simulink model "FinalCircuit"  (R2021b)
settings: Solver=ode4  StartTime=0.0  StopTime=2e-3  FixedStep=5e-10  RelTol=1e-3
values from neighbouring files (symbols this model uses):
  C = D/fs*(Vc-Vbat)/Rout/delVc    (= 1.03597563342e-05)    [Script.m]
  C2 = D2/fs*(Vc2-Vbat2)/Rout2/delVc2    (= 2.79316389763e-06)    [Script.m]
  fs = 250e3    (= 250000)    [Script.m]
  Gcinf = (abs(evalfr(Tuiind,1i*2*pi*fc)))/sqrt(1+(wLv/2/pi/fc)^2)/abs(evalfr(Gfilter,1i*2*pi*fc))    [Script.m]
  Gcinf2 = (abs(evalfr(Tuiind2,1i*2*pi*fc)))/sqrt(1+(wLv2/2/pi/fc)^2)/abs(evalfr(Gfilter,1i*2*pi*fc))    [Script.m]
  Lm = Vc*Dp/delIlm/fs    (= 0.000738946619669)    [Script.m]
  Lm2 = Vc2*Dp2/delIlm2/fs    (= 0.00253168682241)    [Script.m]
  Rin = 100e-3    (= 0.1)    [Script.m]
  Rout = Rin    (= 0.1)    [Script.m]
  Rsense = 5/0.2    (= 25)    [Script.m]
  Rsense2 = 5/0.1    (= 50)    [Script.m]
  Vbat = 3.7    [Script.m]
  Vin = 3.7    [Script.m]
  Vm = 5    [Script.m]
  wLv = 2*pi*fc*tan(75*pi/180)    [Script.m]
  wLv2 = 2*pi*fc*tan(60*pi/180)    [Script.m]
  wpfilter = 2*pi*30e3    (= 188495.559215)    [Script.m]
  wpfilter2 = 2*pi*10e3    (= 62831.8530718)    [Script.m]
libraries: spsCurrentMeasurementLib x25, spsVoltageMeasurementLib x18, spsSeriesRLCBranchLib x12, spsMosfetLib x9, spsLinearTransformerLib x4, simulink x4, spsDCVoltageSourceLib x4, spsDiodeLib x2, spspowerguiLib x2, spsControlledCurrentSourceLib x1
settings Model: SimulationMode=rapid-accelerator  Creator=ee3210698  LastModifiedBy=ee3210698

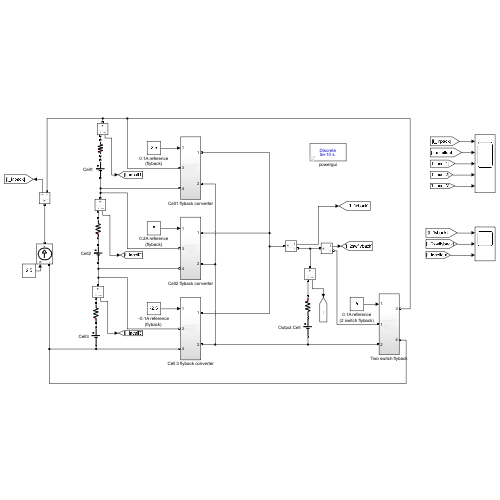
[thumbnail: Simulink's stored preview of the top-level diagram]
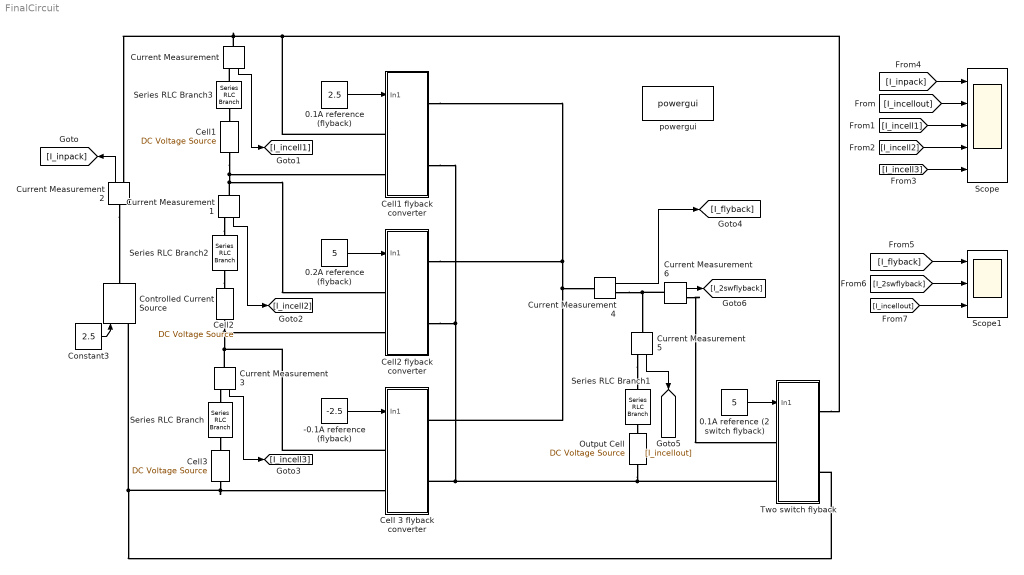
== system FinalCircuit ==
  "-0.1A reference (flyback) " : Constant  Value=-2.5
  0.1A reference (2 switch flyback) : Constant  Value=5
  0.1A reference (flyback) : Constant  Value=2.5
  0.2A reference (flyback) : Constant  Value=5
  Cell 3 flyback converter : Subsystem
  Cell1 : spsDCVoltageSourceLib/DC Voltage Source  Amplitude=Vin  Measurements=None
  Cell1 flyback converter : Subsystem
  Cell2 : spsDCVoltageSourceLib/DC Voltage Source  Amplitude=Vin  Measurements=None
  Cell2 flyback converter : Subsystem
  Cell3 : spsDCVoltageSourceLib/DC Voltage Source  Amplitude=Vin  Measurements=None
  Constant3 : Constant  Value=2.5
  Controlled Current Source : spsControlledCurrentSourceLib/Controlled Current Source  Initialize=on  Source_Type=DC  Amplitude=2.5  Phase=0  Frequency=0  Measurements=None
  Current Measurement{,1..6} (7 alike) : spsCurrentMeasurementLib/Current Measurement  PhasorSimulation=off  OutputType=Complex  PSBequivalent=0
  Output Cell : spsDCVoltageSourceLib/DC Voltage Source  Amplitude=Vbat  Measurements=None
  Scope : Scope  NumInputPorts=5
  Scope1 : Scope  NumInputPorts=3
  Series RLC Branch : spsSeriesRLCBranchLib/Series RLC Branch  LConnTagsString=__new0  RConnTagsString=__new0  BranchType=R  Resistance=Rin  Inductance=1e-3  SetiL0=off  InitialCurrent=0  Capacitance=1e-6  Setx0=off  InitialVoltage=0  Measurements=None
  Series RLC Branch1 : spsSeriesRLCBranchLib/Series RLC Branch  LConnTagsString=__new0  RConnTagsString=__new0  BranchType=R  Resistance=Rout  Inductance=1e-3  SetiL0=off  InitialCurrent=0  Capacitance=1e-6  Setx0=off  InitialVoltage=0  Measurements=None
  Series RLC Branch2 : spsSeriesRLCBranchLib/Series RLC Branch  LConnTagsString=__new0  RConnTagsString=__new0  BranchType=R  Resistance=Rin  Inductance=1e-3  SetiL0=off  InitialCurrent=0  Capacitance=1e-6  Setx0=off  InitialVoltage=0  Measurements=None
  Series RLC Branch3 : spsSeriesRLCBranchLib/Series RLC Branch  LConnTagsString=__new0  RConnTagsString=__new0  BranchType=R  Resistance=Rin  Inductance=1e-3  SetiL0=off  InitialCurrent=0  Capacitance=1e-6  Setx0=off  InitialVoltage=0  Measurements=None
  Two switch flyback : Subsystem
  powergui : spspowerguiLib/powergui  Priority=1  SimulationMode=Discrete  SampleTime=5e-10  frequency=60  Iterations=50  frequencyindice=0  Pbase=100e6  ErrMax=1e-4  UnitsV=kV  UnitsW=MW  buscounter=0  FunctionMessages=off  echomessages=off  EnableUseOfTLC=off  CurrentSourceSwitches=off  DisableSnubberDevices=off  DisableRonSwitches=off  DisableVfSwitches=off  DisplayEquations=off  AutomaticDiscreteSolvers=off  SolverType=Tustin/Backward Euler (TBE)  Interpol=off  ExternalGateDelay=off  methode=off  Ts=100  x0status=blocks  SPID=on  SwTol=0  HookPort=off  NonlinearTolerance=1e-4  nMaxIteration=100  ContinueOnMaxIteration=off  RestoreLinks=warning  ResistiveCurrentMeasurement=off  Frange=[0:2:500]  Ylog=off  Xlog=on  ShowGrid=off  save=off  variable=ZData  structure=0  ZoomFFT=off  StartTime=0.0  cycles=1  DisplayStyle=1  fundamental=60  FreqAxis=off  MaxFrequency=1000  frequencyindicesteady=1  RmsSteady=1  display=off
  wires:
  "-0.1A reference (flyback) "/1 -> Cell 3 flyback converter/1(In1)
  0.2A reference (flyback)/1 -> Cell2 flyback converter/1(In1)
  0.1A reference (flyback)/1 -> Cell1 flyback converter/1(In1)
  Current Measurement2/1 -> [I_inpack]
  Current Measurement1/1 -> [I_incell2]
  Current Measurement3/1 -> [I_incell3]
  Current Measurement4/1 -> [I_flyback]
  [I_incellout] -> Scope/2
  [I_incell1] -> Scope/3
  [I_incell2] -> Scope/4
  [I_incell3] -> Scope/5
  [I_inpack] -> Scope/1
  Constant3/1 -> Controlled Current Source/1
  Current Measurement/1 -> [I_incell1]
  0.1A reference (2 switch flyback)/1 -> Two switch flyback/1(In1)
  Current Measurement5/1 -> [I_incellout]
  [I_flyback] -> Scope1/1
  Current Measurement6/1 -> [I_2swflyback]
  [I_2swflyback] -> Scope1/2
  [I_incellout] -> Scope1/3
  connections:
  Cell3/LConn1 -- Cell 3 flyback converter/LConn2 -- Two switch flyback/RConn2 -- Controlled Current Source/LConn1
  Series RLC Branch/LConn1 -- Cell3/RConn1
  Series RLC Branch1/RConn1 -- Output Cell/RConn1
  Output Cell/LConn1 -- Cell1 flyback converter/RConn2 -- Cell2 flyback converter/RConn2 -- Cell 3 flyback converter/RConn2 -- Two switch flyback/LConn2
  Series RLC Branch2/LConn1 -- Cell2/RConn1
  Cell2/LConn1 -- Cell 3 flyback converter/LConn1 -- Current Measurement3/LConn1 -- Cell2 flyback converter/LConn2
  Cell1/LConn1 -- Cell2 flyback converter/LConn1 -- Current Measurement1/LConn1 -- Cell1 flyback converter/LConn2
  Series RLC Branch3/LConn1 -- Cell1/RConn1
  Cell1 flyback converter/LConn1 -- Current Measurement2/RConn1 -- Current Measurement/LConn1 -- Two switch flyback/RConn1
  Current Measurement2/LConn1 -- Controlled Current Source/RConn1
  Cell1 flyback converter/RConn1 -- Cell 3 flyback converter/RConn1 -- Current Measurement4/LConn1 -- Cell2 flyback converter/RConn1
  Current Measurement4/RConn1 -- Current Measurement6/LConn1 -- Current Measurement5/LConn1
  Series RLC Branch3/RConn1 -- Current Measurement/RConn1
  Current Measurement1/RConn1 -- Series RLC Branch2/RConn1
  Current Measurement3/RConn1 -- Series RLC Branch/RConn1
  Current Measurement5/RConn1 -- Series RLC Branch1/LConn1
  Current Measurement6/RConn1 -- Two switch flyback/LConn1

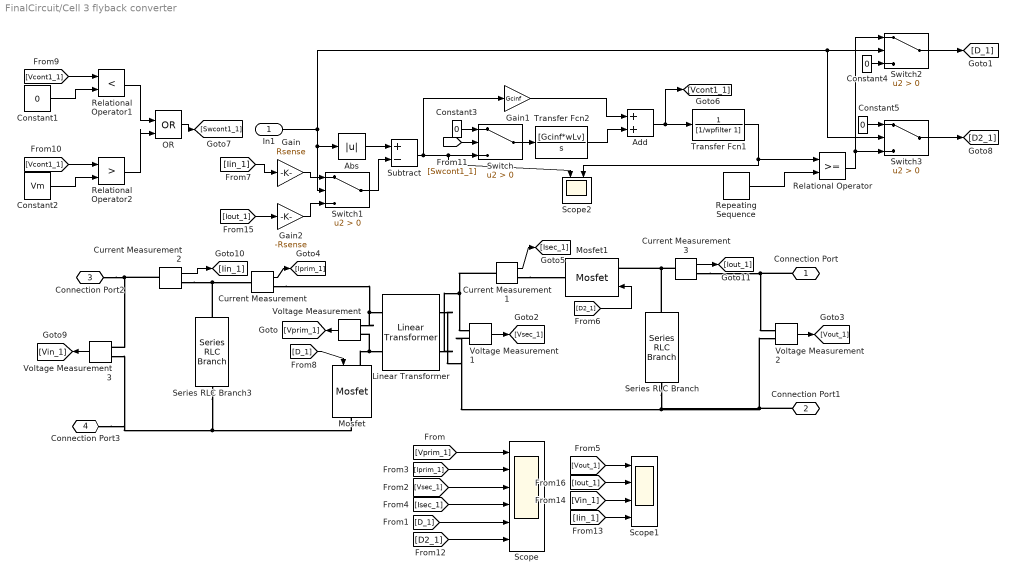
== system FinalCircuit/Cell 3 flyback converter ==
  In1 : Inport
  Abs : Abs
  Add : Sum
  Constant{1,3..5} (4 alike) : Constant  Value=0
  Constant2 : Constant  Value=Vm
  Current Measurement{,1..3} (4 alike) : spsCurrentMeasurementLib/Current Measurement  PhasorSimulation=off  OutputType=Complex  PSBequivalent=0
  Gain : Gain  Gain=Rsense
  Gain1 : Gain  Gain=Gcinf
  Gain2 : Gain  Gain=-Rsense
  Linear Transformer : spsLinearTransformerLib/Linear Transformer  UNITS=SI  NominalPower=[ 200 250e3 ]  winding1=[10 0.1 0]  winding2=[10 0 0]  ThreeWindings=off  winding3=[3.15e+05 0.7938 0.084225]  RmLm=[inf Lm]  Measurements=None  DataType=on
  Mosfet : spsMosfetLib/Mosfet  Ron=0.001  Lon=0  Rd=0.001  Vfd=0  IC=0  Rs=10e9  Cs=inf  Measurements=off
  Mosfet1 : spsMosfetLib/Mosfet  Ron=0.001  Lon=0  Rd=0.001  Vfd=0  IC=0  Rs=10e9  Cs=inf  Measurements=off
  OR : Logic  Operator=OR  IconShape=distinctive  AllPortsSameDT=off  OutDataTypeStr=boolean
  Relational Operator : RelationalOperator  OutDataTypeStr=boolean  RndMeth=Simplest
  Relational Operator1 : RelationalOperator  Operator=<  OutDataTypeStr=boolean  RndMeth=Simplest
  Relational Operator2 : RelationalOperator  Operator=>  OutDataTypeStr=boolean  RndMeth=Simplest
  Repeating Sequence : simulink/Sources/Repeating Sequence  rep_seq_t=[0 1/fs]  rep_seq_y=[0 Vm]
  Scope : Scope  NumInputPorts=6
  Scope1 : Scope  NumInputPorts=4
  Scope2 : Scope  NumInputPorts=2
  Series RLC Branch : spsSeriesRLCBranchLib/Series RLC Branch  LConnTagsString=__new0  RConnTagsString=__new0  BranchType=C  Resistance=1  Inductance=1e-3  SetiL0=off  InitialCurrent=0  Capacitance=C  Setx0=off  InitialVoltage=0  Measurements=None
  Series RLC Branch3 : spsSeriesRLCBranchLib/Series RLC Branch  LConnTagsString=__new0  RConnTagsString=__new0  BranchType=C  Resistance=1  Inductance=1e-3  SetiL0=off  InitialCurrent=0  Capacitance=C  Setx0=off  InitialVoltage=0  Measurements=None
  Subtract : Sum  Inputs=+-
  Switch{,1..3} (4 alike) : Switch  Criteria=u2 > Threshold
  Transfer Fcn1 : TransferFcn  Denominator=[1/wpfilter 1]
  Transfer Fcn2 : TransferFcn  Numerator=[Gcinf*wLv]  Denominator=[1 0]
  Voltage Measurement{,1..3} (4 alike) : spsVoltageMeasurementLib/Voltage Measurement  PhasorSimulation=off  OutputType=Complex  PSBequivalent=0
  Connection Port : PMIOPort  Side=Right
  Connection Port1 : PMIOPort  Port=2  Side=Right
  Connection Port2 : PMIOPort  Port=3  Side=Left
  Connection Port3 : PMIOPort  Port=4  Side=Left
  wires:
  [Iprim_1] -> Scope/2
  Subtract/1 -> Switch/3, Scope2/1, Gain1/1
  Switch1/1 -> Subtract/2
  [Swcont1_1] -> Switch/2
  Constant2/1 -> Relational Operator2/2
  In1/1 -> Switch1/2, Abs/1, Switch3/2, Switch2/2
  Transfer Fcn1/1 -> Scope2/2, Relational Operator/1
  Gain/1 -> Switch1/1
  Current Measurement1/1 -> [Isec_1]
  Relational Operator/1 -> Switch2/1, Switch3/3
  Gain2/1 -> Switch1/3
  OR/1 -> [Swcont1_1]
  Abs/1 -> Subtract/1
  [Vcont1_1] -> Relational Operator2/1
  [Iin_1] -> Scope1/4
  Add/1 -> Transfer Fcn1/1, [Vcont1_1]
  Constant5/1 -> Switch3/1
  Current Measurement/1 -> [Iprim_1]
  [Vin_1] -> Scope1/3
  Constant4/1 -> Switch2/3
  Current Measurement2/1 -> [Iin_1]
  [Vsec_1] -> Scope/3
  [D2_1] -> Mosfet1/1
  [D_1] -> Mosfet/1
  Voltage Measurement3/1 -> [Vin_1]
  [D_1] -> Scope/5
  [Isec_1] -> Scope/4
  Relational Operator2/1 -> OR/2
  Transfer Fcn2/1 -> Add/2
  Constant1/1 -> Relational Operator1/2
  Relational Operator1/1 -> OR/1
  Switch/1 -> Transfer Fcn2/1
  [D2_1] -> Scope/6
  [Vcont1_1] -> Relational Operator1/1
  Switch3/1 -> [D2_1]
  Voltage Measurement/1 -> [Vprim_1]
  [Vout_1] -> Scope1/1
  [Iin_1] -> Gain/1
  [Vprim_1] -> Scope/1
  Current Measurement3/1 -> [Iout_1]
  Voltage Measurement2/1 -> [Vout_1]
  [Iout_1] -> Scope1/2
  Switch2/1 -> [D_1]
  [Iout_1] -> Gain2/1
  Gain1/1 -> Add/1
  Voltage Measurement1/1 -> [Vsec_1]
  Repeating Sequence/1 -> Relational Operator/2
  Constant3/1 -> Switch/1
  connections:
  Current Measurement3/LConn1 -- Series RLC Branch/LConn1 -- Mosfet1/LConn1
  Series RLC Branch/RConn1 -- Linear Transformer/RConn1 -- Voltage Measurement1/LConn1 -- Voltage Measurement2/LConn2 -- Connection Port1/RConn1
  Linear Transformer/RConn2 -- Current Measurement1/LConn1 -- Voltage Measurement1/LConn2
  Series RLC Branch3/RConn1 -- Connection Port3/RConn1 -- Voltage Measurement3/LConn2 -- Mosfet/RConn1
  Linear Transformer/LConn2 -- Mosfet/LConn1 -- Voltage Measurement/LConn2
  Current Measurement1/RConn1 -- Mosfet1/RConn1
  Current Measurement2/LConn1 -- Voltage Measurement3/LConn1 -- Connection Port2/RConn1
  Current Measurement3/RConn1 -- Voltage Measurement2/LConn1 -- Connection Port/RConn1
  Linear Transformer/LConn1 -- Voltage Measurement/LConn1 -- Current Measurement/RConn1
  Current Measurement2/RConn1 -- Series RLC Branch3/LConn1 -- Current Measurement/LConn1

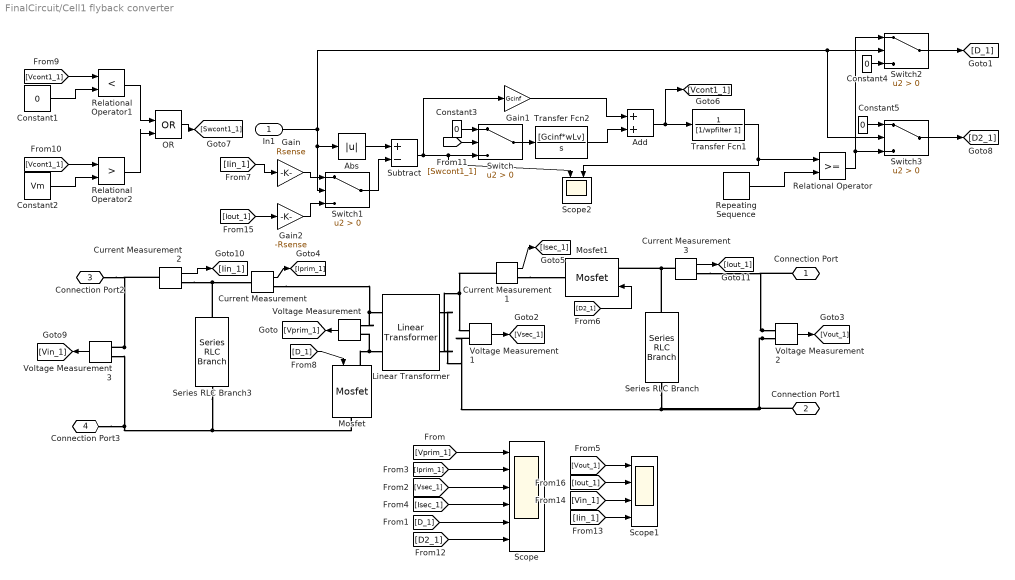
== system FinalCircuit/Cell1 flyback converter ==
  In1 : Inport
  Abs : Abs
  Add : Sum
  Constant{1,3..5} (4 alike) : Constant  Value=0
  Constant2 : Constant  Value=Vm
  Current Measurement{,1..3} (4 alike) : spsCurrentMeasurementLib/Current Measurement  PhasorSimulation=off  OutputType=Complex  PSBequivalent=0
  Gain : Gain  Gain=Rsense
  Gain1 : Gain  Gain=Gcinf
  Gain2 : Gain  Gain=-Rsense
  Linear Transformer : spsLinearTransformerLib/Linear Transformer  UNITS=SI  NominalPower=[ 200 250e3 ]  winding1=[10 0.1 0]  winding2=[10 0 0]  ThreeWindings=off  winding3=[3.15e+05 0.7938 0.084225]  RmLm=[inf Lm]  Measurements=None  DataType=on
  Mosfet : spsMosfetLib/Mosfet  Ron=0.001  Lon=0  Rd=0.001  Vfd=0  IC=0  Rs=10e9  Cs=inf  Measurements=off
  Mosfet1 : spsMosfetLib/Mosfet  Ron=0.001  Lon=0  Rd=0.001  Vfd=0  IC=0  Rs=10e9  Cs=inf  Measurements=off
  OR : Logic  Operator=OR  IconShape=distinctive  AllPortsSameDT=off  OutDataTypeStr=boolean
  Relational Operator : RelationalOperator  OutDataTypeStr=boolean  RndMeth=Simplest
  Relational Operator1 : RelationalOperator  Operator=<  OutDataTypeStr=boolean  RndMeth=Simplest
  Relational Operator2 : RelationalOperator  Operator=>  OutDataTypeStr=boolean  RndMeth=Simplest
  Repeating Sequence : simulink/Sources/Repeating Sequence  rep_seq_t=[0 1/fs]  rep_seq_y=[0 Vm]
  Scope : Scope  NumInputPorts=6
  Scope1 : Scope  NumInputPorts=4
  Scope2 : Scope  NumInputPorts=2
  Series RLC Branch : spsSeriesRLCBranchLib/Series RLC Branch  LConnTagsString=__new0  RConnTagsString=__new0  BranchType=C  Resistance=1  Inductance=1e-3  SetiL0=off  InitialCurrent=0  Capacitance=C  Setx0=off  InitialVoltage=0  Measurements=None
  Series RLC Branch3 : spsSeriesRLCBranchLib/Series RLC Branch  LConnTagsString=__new0  RConnTagsString=__new0  BranchType=C  Resistance=1  Inductance=1e-3  SetiL0=off  InitialCurrent=0  Capacitance=C  Setx0=off  InitialVoltage=0  Measurements=None
  Subtract : Sum  Inputs=+-
  Switch{,1..3} (4 alike) : Switch  Criteria=u2 > Threshold
  Transfer Fcn1 : TransferFcn  Denominator=[1/wpfilter 1]
  Transfer Fcn2 : TransferFcn  Numerator=[Gcinf*wLv]  Denominator=[1 0]
  Voltage Measurement{,1..3} (4 alike) : spsVoltageMeasurementLib/Voltage Measurement  PhasorSimulation=off  OutputType=Complex  PSBequivalent=0
  Connection Port : PMIOPort  Side=Right
  Connection Port1 : PMIOPort  Port=2  Side=Right
  Connection Port2 : PMIOPort  Port=3  Side=Left
  Connection Port3 : PMIOPort  Port=4  Side=Left
  wires:
  Constant3/1 -> Switch/1
  Repeating Sequence/1 -> Relational Operator/2
  Voltage Measurement1/1 -> [Vsec_1]
  Gain1/1 -> Add/1
  [Iout_1] -> Gain2/1
  Switch2/1 -> [D_1]
  [Iout_1] -> Scope1/2
  Voltage Measurement2/1 -> [Vout_1]
  Current Measurement3/1 -> [Iout_1]
  [Vprim_1] -> Scope/1
  [Iin_1] -> Gain/1
  [Vout_1] -> Scope1/1
  Voltage Measurement/1 -> [Vprim_1]
  Switch3/1 -> [D2_1]
  [Vcont1_1] -> Relational Operator1/1
  [D2_1] -> Scope/6
  Switch/1 -> Transfer Fcn2/1
  Relational Operator1/1 -> OR/1
  Constant1/1 -> Relational Operator1/2
  Transfer Fcn2/1 -> Add/2
  Relational Operator2/1 -> OR/2
  [Isec_1] -> Scope/4
  [D_1] -> Scope/5
  Voltage Measurement3/1 -> [Vin_1]
  [D_1] -> Mosfet/1
  [D2_1] -> Mosfet1/1
  [Vsec_1] -> Scope/3
  Current Measurement2/1 -> [Iin_1]
  Constant4/1 -> Switch2/3
  [Vin_1] -> Scope1/3
  Current Measurement/1 -> [Iprim_1]
  Constant5/1 -> Switch3/1
  Add/1 -> [Vcont1_1], Transfer Fcn1/1
  [Iin_1] -> Scope1/4
  [Vcont1_1] -> Relational Operator2/1
  Abs/1 -> Subtract/1
  OR/1 -> [Swcont1_1]
  Gain2/1 -> Switch1/3
  Relational Operator/1 -> Switch3/3, Switch2/1
  Current Measurement1/1 -> [Isec_1]
  Gain/1 -> Switch1/1
  Transfer Fcn1/1 -> Relational Operator/1, Scope2/2
  In1/1 -> Switch2/2, Switch3/2, Abs/1, Switch1/2
  Constant2/1 -> Relational Operator2/2
  [Swcont1_1] -> Switch/2
  Switch1/1 -> Subtract/2
  Subtract/1 -> Gain1/1, Scope2/1, Switch/3
  [Iprim_1] -> Scope/2
  connections:
  Series RLC Branch3/LConn1 -- Current Measurement2/RConn1 -- Current Measurement/LConn1
  Voltage Measurement/LConn1 -- Linear Transformer/LConn1 -- Current Measurement/RConn1
  Voltage Measurement2/LConn1 -- Connection Port/RConn1 -- Current Measurement3/RConn1
  Voltage Measurement3/LConn1 -- Current Measurement2/LConn1 -- Connection Port2/RConn1
  Current Measurement1/RConn1 -- Mosfet1/RConn1
  Mosfet/LConn1 -- Linear Transformer/LConn2 -- Voltage Measurement/LConn2
  Voltage Measurement3/LConn2 -- Connection Port3/RConn1 -- Series RLC Branch3/RConn1 -- Mosfet/RConn1
  Current Measurement1/LConn1 -- Linear Transformer/RConn2 -- Voltage Measurement1/LConn2
  Voltage Measurement2/LConn2 -- Connection Port1/RConn1 -- Voltage Measurement1/LConn1 -- Linear Transformer/RConn1 -- Series RLC Branch/RConn1
  Series RLC Branch/LConn1 -- Current Measurement3/LConn1 -- Mosfet1/LConn1

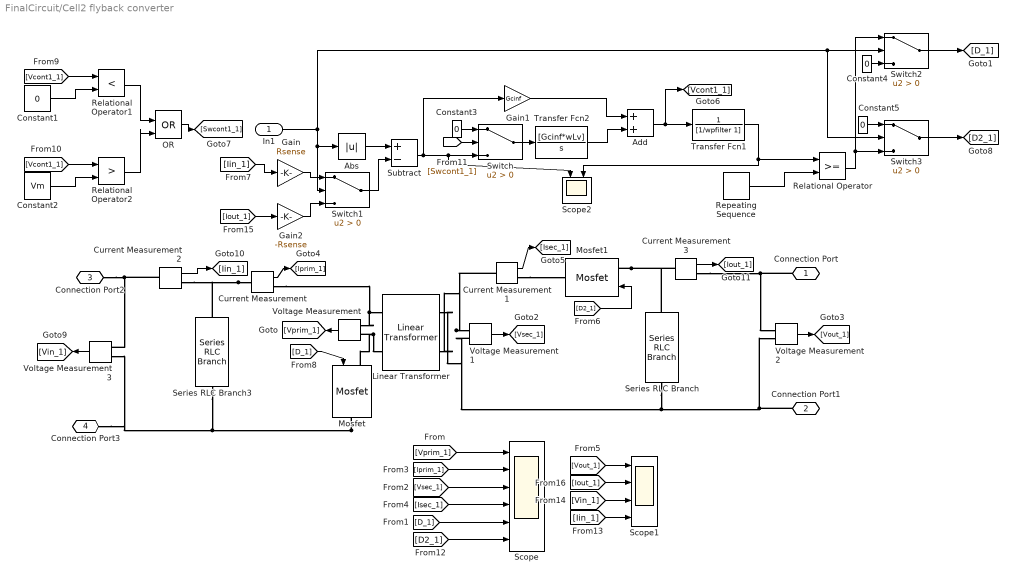
== system FinalCircuit/Cell2 flyback converter ==
  In1 : Inport
  Abs : Abs
  Add : Sum
  Constant{1,3..5} (4 alike) : Constant  Value=0
  Constant2 : Constant  Value=Vm
  Current Measurement{,1..3} (4 alike) : spsCurrentMeasurementLib/Current Measurement  PhasorSimulation=off  OutputType=Complex  PSBequivalent=0
  Gain : Gain  Gain=Rsense
  Gain1 : Gain  Gain=Gcinf
  Gain2 : Gain  Gain=-Rsense
  Linear Transformer : spsLinearTransformerLib/Linear Transformer  UNITS=SI  NominalPower=[ 200 250e3 ]  winding1=[10 0.1 0]  winding2=[10 0 0]  ThreeWindings=off  winding3=[3.15e+05 0.7938 0.084225]  RmLm=[inf Lm]  Measurements=None  DataType=on
  Mosfet : spsMosfetLib/Mosfet  Ron=0.001  Lon=0  Rd=0.001  Vfd=0  IC=0  Rs=10e9  Cs=inf  Measurements=off
  Mosfet1 : spsMosfetLib/Mosfet  Ron=0.001  Lon=0  Rd=0.001  Vfd=0  IC=0  Rs=10e9  Cs=inf  Measurements=off
  OR : Logic  Operator=OR  IconShape=distinctive  AllPortsSameDT=off  OutDataTypeStr=boolean
  Relational Operator : RelationalOperator  OutDataTypeStr=boolean  RndMeth=Simplest
  Relational Operator1 : RelationalOperator  Operator=<  OutDataTypeStr=boolean  RndMeth=Simplest
  Relational Operator2 : RelationalOperator  Operator=>  OutDataTypeStr=boolean  RndMeth=Simplest
  Repeating Sequence : simulink/Sources/Repeating Sequence  rep_seq_t=[0 1/fs]  rep_seq_y=[0 Vm]
  Scope : Scope  NumInputPorts=6
  Scope1 : Scope  NumInputPorts=4
  Scope2 : Scope  NumInputPorts=2
  Series RLC Branch : spsSeriesRLCBranchLib/Series RLC Branch  LConnTagsString=__new0  RConnTagsString=__new0  BranchType=C  Resistance=1  Inductance=1e-3  SetiL0=off  InitialCurrent=0  Capacitance=C  Setx0=off  InitialVoltage=0  Measurements=None
  Series RLC Branch3 : spsSeriesRLCBranchLib/Series RLC Branch  LConnTagsString=__new0  RConnTagsString=__new0  BranchType=C  Resistance=1  Inductance=1e-3  SetiL0=off  InitialCurrent=0  Capacitance=C  Setx0=off  InitialVoltage=0  Measurements=None
  Subtract : Sum  Inputs=+-
  Switch{,1..3} (4 alike) : Switch  Criteria=u2 > Threshold
  Transfer Fcn1 : TransferFcn  Denominator=[1/wpfilter 1]
  Transfer Fcn2 : TransferFcn  Numerator=[Gcinf*wLv]  Denominator=[1 0]
  Voltage Measurement{,1..3} (4 alike) : spsVoltageMeasurementLib/Voltage Measurement  PhasorSimulation=off  OutputType=Complex  PSBequivalent=0
  Connection Port : PMIOPort  Side=Right
  Connection Port1 : PMIOPort  Port=2  Side=Right
  Connection Port2 : PMIOPort  Port=3  Side=Left
  Connection Port3 : PMIOPort  Port=4  Side=Left
  wires:
  [Iprim_1] -> Scope/2
  Subtract/1 -> Switch/3, Scope2/1, Gain1/1
  Switch1/1 -> Subtract/2
  [Swcont1_1] -> Switch/2
  Constant2/1 -> Relational Operator2/2
  In1/1 -> Switch1/2, Abs/1, Switch3/2, Switch2/2
  Transfer Fcn1/1 -> Scope2/2, Relational Operator/1
  Gain/1 -> Switch1/1
  Current Measurement1/1 -> [Isec_1]
  Relational Operator/1 -> Switch2/1, Switch3/3
  Gain2/1 -> Switch1/3
  OR/1 -> [Swcont1_1]
  Abs/1 -> Subtract/1
  [Vcont1_1] -> Relational Operator2/1
  [Iin_1] -> Scope1/4
  Add/1 -> Transfer Fcn1/1, [Vcont1_1]
  Constant5/1 -> Switch3/1
  Current Measurement/1 -> [Iprim_1]
  [Vin_1] -> Scope1/3
  Constant4/1 -> Switch2/3
  Current Measurement2/1 -> [Iin_1]
  [Vsec_1] -> Scope/3
  [D2_1] -> Mosfet1/1
  [D_1] -> Mosfet/1
  Voltage Measurement3/1 -> [Vin_1]
  [D_1] -> Scope/5
  [Isec_1] -> Scope/4
  Relational Operator2/1 -> OR/2
  Transfer Fcn2/1 -> Add/2
  Constant1/1 -> Relational Operator1/2
  Relational Operator1/1 -> OR/1
  Switch/1 -> Transfer Fcn2/1
  [D2_1] -> Scope/6
  [Vcont1_1] -> Relational Operator1/1
  Switch3/1 -> [D2_1]
  Voltage Measurement/1 -> [Vprim_1]
  [Vout_1] -> Scope1/1
  [Iin_1] -> Gain/1
  [Vprim_1] -> Scope/1
  Current Measurement3/1 -> [Iout_1]
  Voltage Measurement2/1 -> [Vout_1]
  [Iout_1] -> Scope1/2
  Switch2/1 -> [D_1]
  [Iout_1] -> Gain2/1
  Gain1/1 -> Add/1
  Voltage Measurement1/1 -> [Vsec_1]
  Repeating Sequence/1 -> Relational Operator/2
  Constant3/1 -> Switch/1
  connections:
  Mosfet1/LConn1 -- Current Measurement3/LConn1 -- Series RLC Branch/LConn1
  Series RLC Branch/RConn1 -- Linear Transformer/RConn1 -- Voltage Measurement1/LConn1 -- Connection Port1/RConn1 -- Voltage Measurement2/LConn2
  Voltage Measurement1/LConn2 -- Linear Transformer/RConn2 -- Current Measurement1/LConn1
  Mosfet/RConn1 -- Series RLC Branch3/RConn1 -- Connection Port3/RConn1 -- Voltage Measurement3/LConn2
  Voltage Measurement/LConn2 -- Linear Transformer/LConn2 -- Mosfet/LConn1
  Current Measurement1/RConn1 -- Mosfet1/RConn1
  Connection Port2/RConn1 -- Current Measurement2/LConn1 -- Voltage Measurement3/LConn1
  Current Measurement3/RConn1 -- Connection Port/RConn1 -- Voltage Measurement2/LConn1
  Current Measurement/RConn1 -- Linear Transformer/LConn1 -- Voltage Measurement/LConn1
  Current Measurement/LConn1 -- Current Measurement2/RConn1 -- Series RLC Branch3/LConn1

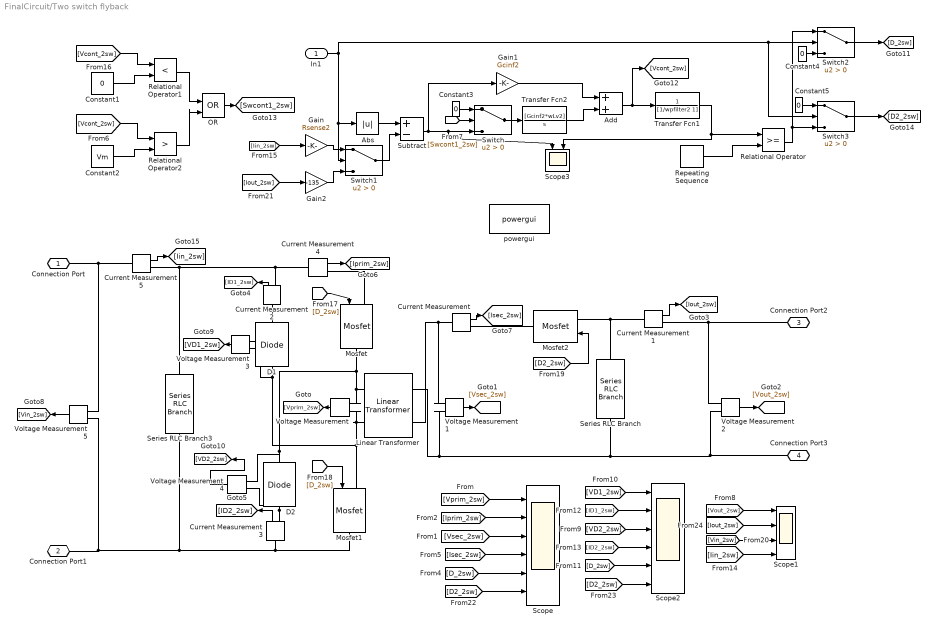
== system FinalCircuit/Two switch flyback ==
  In1 : Inport
  Abs : Abs
  Add : Sum
  Constant{1,3..5} (4 alike) : Constant  Value=0
  Constant2 : Constant  Value=Vm
  Current Measurement{,1..5} (6 alike) : spsCurrentMeasurementLib/Current Measurement  PhasorSimulation=off  OutputType=Complex  PSBequivalent=0
  D1 : spsDiodeLib/Diode  Ron=0.001  Lon=0  Vf=0  IC=0  UseSnubber=0  Rs=inf  Cs=inf  Measurements=off
  D2 : spsDiodeLib/Diode  Ron=0.001  Lon=0  Vf=0  IC=0  UseSnubber=0  Rs=inf  Cs=inf  Measurements=off
  Gain : Gain  Gain=Rsense2
  Gain1 : Gain  Gain=Gcinf2
  Gain2 : Gain  Gain=-135
  Linear Transformer : spsLinearTransformerLib/Linear Transformer  UNITS=SI  NominalPower=[ 200 fs ]  winding1=[10 0 0]  winding2=[40 0 0]  ThreeWindings=off  winding3=[3.15e+05 0.7938 0.084225]  RmLm=[inf Lm2]  Measurements=None  DataType=on
  Mosfet : spsMosfetLib/Mosfet  Ron=0.001  Lon=0  Rd=0.001  Vfd=0  IC=0  Rs=1e9  Cs=inf  Measurements=off
  Mosfet1 : spsMosfetLib/Mosfet  Ron=0.1  Lon=0  Rd=0.01  Vfd=0  IC=0  Rs=1e9  Cs=inf  Measurements=off
  Mosfet2 : spsMosfetLib/Mosfet  Ron=0.1  Lon=0  Rd=0.01  Vfd=0  IC=0  Rs=1e9  Cs=inf  Measurements=off
  OR : Logic  Operator=OR  IconShape=distinctive  AllPortsSameDT=off  OutDataTypeStr=boolean
  Relational Operator : RelationalOperator  OutDataTypeStr=boolean  RndMeth=Simplest
  Relational Operator1 : RelationalOperator  Operator=<  OutDataTypeStr=boolean  RndMeth=Simplest
  Relational Operator2 : RelationalOperator  Operator=>  OutDataTypeStr=boolean  RndMeth=Simplest
  Repeating Sequence : simulink/Sources/Repeating Sequence  rep_seq_t=[0 1/fs]  rep_seq_y=[0 Vm]
  Scope : Scope  NumInputPorts=6
  Scope1 : Scope  NumInputPorts=4
  Scope2 : Scope  NumInputPorts=6
  Scope3 : Scope  NumInputPorts=2
  Series RLC Branch : spsSeriesRLCBranchLib/Series RLC Branch  LConnTagsString=__new0  RConnTagsString=__new0  BranchType=C  Resistance=1  Inductance=1e-3  SetiL0=off  InitialCurrent=0  Capacitance=C2  Setx0=off  InitialVoltage=0  Measurements=None
  Series RLC Branch3 : spsSeriesRLCBranchLib/Series RLC Branch  LConnTagsString=__new0  RConnTagsString=__new0  BranchType=C  Resistance=1  Inductance=1e-3  SetiL0=off  InitialCurrent=0  Capacitance=C2*3  Setx0=off  InitialVoltage=0  Measurements=None
  Subtract : Sum  Inputs=+-
  Switch{,1..3} (4 alike) : Switch  Criteria=u2 > Threshold
  Transfer Fcn1 : TransferFcn  Denominator=[1/wpfilter2 1]
  Transfer Fcn2 : TransferFcn  Numerator=[Gcinf2*wLv2]  Denominator=[1 0]
  Voltage Measurement{,1..5} (6 alike) : spsVoltageMeasurementLib/Voltage Measurement  PhasorSimulation=off  OutputType=Complex  PSBequivalent=0
  powergui : spspowerguiLib/powergui  Priority=1  SimulationMode=Discrete  SampleTime=5e-10  frequency=60  Iterations=50  frequencyindice=0  Pbase=100e6  ErrMax=1e-4  UnitsV=kV  UnitsW=MW  buscounter=0  FunctionMessages=off  echomessages=off  EnableUseOfTLC=off  CurrentSourceSwitches=off  DisableSnubberDevices=off  DisableRonSwitches=off  DisableVfSwitches=off  DisplayEquations=off  AutomaticDiscreteSolvers=off  SolverType=Tustin/Backward Euler (TBE)  Interpol=off  ExternalGateDelay=off  methode=off  Ts=100  x0status=blocks  SPID=on  SwTol=0  HookPort=off  NonlinearTolerance=1e-4  nMaxIteration=100  ContinueOnMaxIteration=off  RestoreLinks=warning  ResistiveCurrentMeasurement=off  Frange=[0:2:500]  Ylog=off  Xlog=on  ShowGrid=off  save=off  variable=ZData  structure=0  ZoomFFT=off  StartTime=0.0  cycles=1  DisplayStyle=1  fundamental=60  FreqAxis=off  MaxFrequency=1000  frequencyindicesteady=1  RmsSteady=1  display=off
  Connection Port : PMIOPort  Side=Left
  Connection Port1 : PMIOPort  Port=2  Side=Left
  Connection Port2 : PMIOPort  Port=3  Side=Right
  Connection Port3 : PMIOPort  Port=4  Side=Right
  wires:
  [ID1_2sw] -> Scope2/2
  Switch/1 -> Transfer Fcn2/1
  Switch2/1 -> [D_2sw]
  [D2_2sw] -> Scope/6
  [Iout_2sw] -> Scope1/2
  [Iin_2sw] -> Scope1/4
  Current Measurement1/1 -> [Iout_2sw]
  Voltage Measurement5/1 -> [Vin_2sw]
  [Iprim_2sw] -> Scope/2
  [Iin_2sw] -> Gain/1
  [Vsec_2sw] -> Scope/3
  Gain2/1 -> Switch1/3
  [D_2sw] -> Scope/5
  Current Measurement5/1 -> [Iin_2sw]
  Add/1 -> Transfer Fcn1/1, [Vcont_2sw]
  Gain/1 -> Switch1/1
  [Vin_2sw] -> Scope1/3
  Switch3/1 -> [D2_2sw]
  [Iout_2sw] -> Gain2/1
  [D2_2sw] -> Scope2/6
  In1/1 -> Switch1/2, Abs/1, Switch3/2, Switch2/2
  [Isec_2sw] -> Scope/4
  Gain1/1 -> Add/1
  Constant5/1 -> Switch3/1
  Voltage Measurement1/1 -> [Vsec_2sw]
  [D2_2sw] -> Mosfet2/1
  [Vout_2sw] -> Scope1/1
  Constant3/1 -> Switch/1
  Voltage Measurement/1 -> [Vprim_2sw]
  [Vcont_2sw] -> Relational Operator1/1
  Transfer Fcn1/1 -> Scope3/2, Relational Operator/1
  Relational Operator/1 -> Switch2/1, Switch3/3
  Constant1/1 -> Relational Operator1/2
  Relational Operator2/1 -> OR/2
  Subtract/1 -> Switch/3, Scope3/1, Gain1/1
  [Vprim_2sw] -> Scope/1
  [Vcont_2sw] -> Relational Operator2/1
  [VD2_2sw] -> Scope2/3
  Current Measurement/1 -> [Isec_2sw]
  Abs/1 -> Subtract/1
  Current Measurement2/1 -> [ID1_2sw]
  [Swcont1_2sw] -> Switch/2
  OR/1 -> [Swcont1_2sw]
  [D_2sw] -> Scope2/5
  [VD1_2sw] -> Scope2/1
  [D_2sw] -> Mosfet/1
  Repeating Sequence/1 -> Relational Operator/2
  Constant2/1 -> Relational Operator2/2
  Voltage Measurement2/1 -> [Vout_2sw]
  Current Measurement4/1 -> [Iprim_2sw]
  [D_2sw] -> Mosfet1/1
  Relational Operator1/1 -> OR/1
  Transfer Fcn2/1 -> Add/2
  Constant4/1 -> Switch2/3
  Current Measurement3/1 -> [ID2_2sw]
  Switch1/1 -> Subtract/2
  [ID2_2sw] -> Scope2/4
  Voltage Measurement4/1 -> [VD2_2sw]
  Voltage Measurement3/1 -> [VD1_2sw]
  connections:
  Series RLC Branch/LConn1 -- Mosfet2/LConn1 -- Current Measurement1/LConn1
  Current Measurement5/LConn1 -- Voltage Measurement5/LConn1 -- Connection Port/RConn1
  Voltage Measurement4/LConn2 -- Current Measurement3/RConn1 -- D2/LConn1
  Series RLC Branch/RConn1 -- Linear Transformer/RConn1 -- Voltage Measurement1/LConn2 -- Connection Port3/RConn1 -- Voltage Measurement2/LConn2
  Voltage Measurement3/LConn1 -- Current Measurement2/LConn1 -- D1/RConn1
  Voltage Measurement1/LConn1 -- Linear Transformer/RConn2 -- Current Measurement/LConn1
  Series RLC Branch3/RConn1 -- Voltage Measurement5/LConn2 -- Connection Port1/RConn1 -- Mosfet1/RConn1 -- Current Measurement3/LConn1
  Current Measurement1/RConn1 -- Connection Port2/RConn1 -- Voltage Measurement2/LConn1
  Mosfet1/LConn1 -- Linear Transformer/LConn2 -- Voltage Measurement/LConn2 -- Voltage Measurement3/LConn2 -- D1/LConn1
  Mosfet/RConn1 -- Voltage Measurement/LConn1 -- Linear Transformer/LConn1 -- Voltage Measurement4/LConn1 -- D2/RConn1
  Current Measurement4/LConn1 -- Current Measurement2/RConn1 -- Series RLC Branch3/LConn1 -- Current Measurement5/RConn1
  Current Measurement/RConn1 -- Mosfet2/RConn1
  Current Measurement4/RConn1 -- Mosfet/LConn1
